simulink model "Nonlinear_Hinf"  (R2024b)
settings: Solver=VariableStepAuto  StartTime=0.0  StopTime=30  RelTol=1e-3
values from neighbouring files (symbols this model uses):
  Anom = A.NominalValue    [Parameter_CSI.m]
  Bnom = B.NominalValue    [Parameter_CSI.m]
  C = [(b_true*(R_rear/L)^2-a_true*(R_rear^2))*phi_dot*psi_dot*sin(psi)*cos(psi)+c_phi*phi_dot; -Ipz*(R_rear/L)*phi_dot*psi_dot*cos(psi)+c_psi*psi_dot]    [Dynamics_CSI.m]    (also in Parameter_CSI.m = [1 0 0 0 0;0 0 1 0 0])
  D = append(d1,d1,tf(eye(2)),tf(eye(2)))    [D_K_controller2_FINAL.m]    (also in Parameter_CSI.m = zeros(2,2))
  G_tau_phi_nom_tf = minreal(tf(G_tau_phi_nom))    [Parameter_CSI.m]
  G_tau_psi_nom_tf = minreal(tf(G_tau_psi_nom))    [Parameter_CSI.m]
  K_mix = (K_mix)    [Hinf_controller_FINAL.m]
  Rp_nom = R_rear_nom    (= 0.3)    [Parameter_CSI.m]
  u_eq = [c_phi*vx/R_rear_nom; 0]    [Parameter_CSI.m]
  vx = 1    [Dynamics_CSI.m]    (also in Parameter_CSI.m)
  x_eq = [0; 0; vx/R_rear_nom; 0; 0]    [Parameter_CSI.m]
settings Model: Creator=alebe  LastModifiedBy=rober

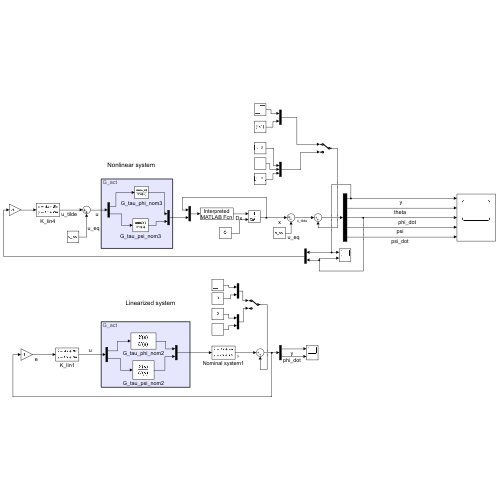
[thumbnail: Simulink's stored preview of the top-level diagram]
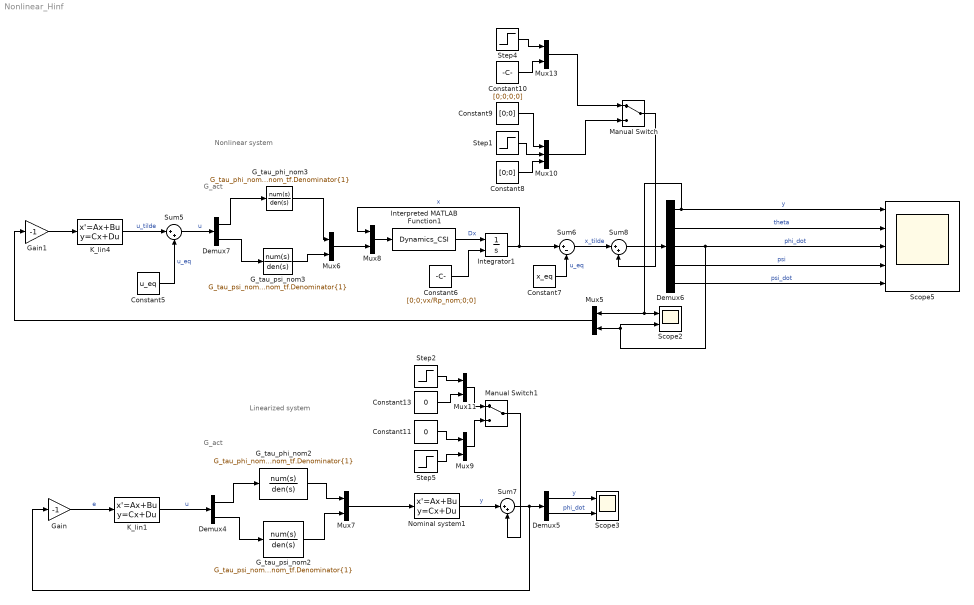
== system Nonlinear_Hinf ==
  note: G_act
  note: Linearized system
  note: G_act
  note: Nonlinear system
  Constant10 : Constant  Value=[0;0;0;0]
  Constant11 : Constant  Value=0
  Constant13 : Constant  Value=0
  Constant5 : Constant  Value=u_eq
  Constant6 : Constant  Value=[0;0;vx/Rp_nom;0;0]
  Constant7 : Constant  Value=x_eq
  Constant8 : Constant  Value=[0;0]
  Constant9 : Constant  Value=[0;0]
  Demux4 : Demux  Outputs=2
  Demux5 : Demux  Outputs=2
  Demux6 : Demux  Outputs=5
  Demux7 : Demux  Outputs=2
  G_tau_phi_nom2 : TransferFcn  Numerator=G_tau_phi_nom_tf.Numerator{1}  Denominator=G_tau_phi_nom_tf.Denominator{1}
  G_tau_phi_nom3 : TransferFcn  Numerator=G_tau_phi_nom_tf.Numerator{1}  Denominator=G_tau_phi_nom_tf.Denominator{1}
  G_tau_psi_nom2 : TransferFcn  Numerator=G_tau_psi_nom_tf.Numerator{1}  Denominator=G_tau_psi_nom_tf.Denominator{1}
  G_tau_psi_nom3 : TransferFcn  Numerator=G_tau_psi_nom_tf.Numerator{1}  Denominator=G_tau_psi_nom_tf.Denominator{1}
  Gain : Gain  Gain=-1
  Gain1 : Gain  Gain=-1
  Integrator1 : Integrator  InitialConditionSource=external
  Interpreted MATLAB Function1 : MATLABFcn  MATLABFcn=Dynamics_CSI
  K_lin1 : StateSpace  A=K_mix.A  B=K_mix.B  C=K_mix.C  D=K_mix.D  InitialCondition=0
  K_lin4 : StateSpace  A=K_mix.A  B=K_mix.B  C=K_mix.C  D=K_mix.D  InitialCondition=0
  Manual Switch : ManualSwitch
  Manual Switch1 : ManualSwitch
  Mux10 : Mux  Inputs=3
  Mux{5..9,11,13} (7 alike) : Mux  Inputs=2
  Nominal system1 : StateSpace  A=Anom  B=Bnom  C=C  D=D  InitialCondition=[0;0;0;0;0]
  Scope2 : Scope  NumInputPorts=2
  Scope3 : Scope  NumInputPorts=2
  Scope5 : Scope  NumInputPorts=5
  Step1 : Step  After=5  SampleTime=0
  Step2 : Step  SampleTime=0
  Step4 : Step  After=1.8  SampleTime=0
  Step5 : Step  SampleTime=0
  Sum5 : Sum  Inputs=|++
  Sum6 : Sum  Inputs=|+-
  Sum7 : Sum  Inputs=|++
  Sum8 : Sum  Inputs=|++
  wires:
  K_lin1/1 -> Demux4/1  "u"
  Gain/1 -> K_lin1/1  "e"
  Step4/1 -> Mux13/1
  Mux5/1 -> Gain1/1
  Demux5/1 -> Scope3/1  "y"
  Constant6/1 -> Integrator1/2
  Mux6/1 -> Mux8/2
  Demux6/3 -> Scope5/3, Scope2/2, Mux5/2  "phi_dot"
  G_tau_phi_nom2/1 -> Mux7/1
  G_tau_psi_nom2/1 -> Mux7/2
  G_tau_psi_nom3/1 -> Mux6/2
  Mux8/1 -> Interpreted MATLAB Function1/1
  Sum5/1 -> Demux7/1  "u"
  Demux5/2 -> Scope3/2  "phi_dot"
  Demux7/1 -> G_tau_phi_nom3/1
  Demux6/4 -> Scope5/4  "psi"
  Constant7/1 -> Sum6/2  "u_eq"
  Demux6/1 -> Mux5/1, Scope2/1, Scope5/1  "y"
  Constant5/1 -> Sum5/2  "u_eq"
  Demux6/5 -> Scope5/5  "psi_dot"
  Gain1/1 -> K_lin4/1
  Demux4/1 -> G_tau_phi_nom2/1
  K_lin4/1 -> Sum5/1  "u_tilde"
  Mux7/1 -> Nominal system1/1
  Sum6/1 -> Sum8/1  "x_tilde"
  Integrator1/1 -> Mux8/1, Sum6/1  "x"
  Sum8/1 -> Demux6/1
  Constant10/1 -> Mux13/2
  Demux7/2 -> G_tau_psi_nom3/1
  Nominal system1/1 -> Sum7/1  "y"
  Demux4/2 -> G_tau_psi_nom2/1
  Sum7/1 -> Gain/1, Demux5/1
  Manual Switch1/1 -> Sum7/2
  Mux13/1 -> Manual Switch/1
  G_tau_phi_nom3/1 -> Mux6/1
  Step5/1 -> Mux9/2
  Demux6/2 -> Scope5/2  "theta"
  Interpreted MATLAB Function1/1 -> Integrator1/1  "Dx"
  Manual Switch/1 -> Sum8/2
  Constant8/1 -> Mux10/3
  Step1/1 -> Mux10/2
  Mux10/1 -> Manual Switch/2
  Constant9/1 -> Mux10/1
  Constant13/1 -> Mux11/2
  Mux11/1 -> Manual Switch1/1
  Step2/1 -> Mux11/1
  Mux9/1 -> Manual Switch1/2
  Constant11/1 -> Mux9/1
